simulink model "Actuatorsim"  (R2023a)
settings: Solver=FixedStepAuto  StartTime=0.0  StopTime=tf  FixedStep=tstep  RelTol=1e-3
values from neighbouring files (symbols this model uses):
  a_ol = [1 2*zeta*wn wn^2]    [ActuatorModel.m]
  b_ol = K*wn^2    (= 6103.86868538)    [ActuatorModel.m]
  k = 55    [ActuatorModel.m]    (also in SysID.m = 11.93; Translational.m = -inv(R)*Bbar'*P)
  p = -800    [ActuatorModel.m]
  z = -375    [ActuatorModel.m]
libraries: simulink x3, simulink_extras x1
settings Model: Creator=Nathan Dablain  LastModifiedBy=Nathan Dablain

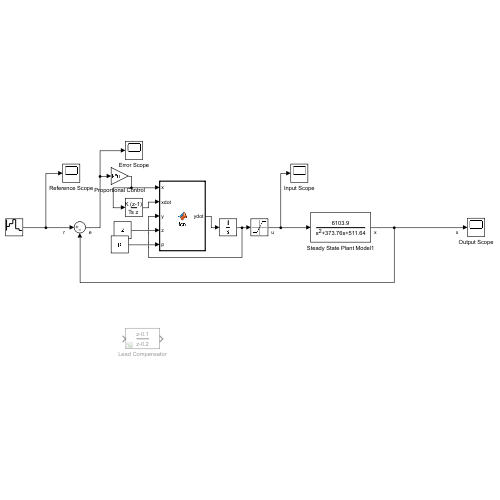
[thumbnail: Simulink's stored preview of the top-level diagram]
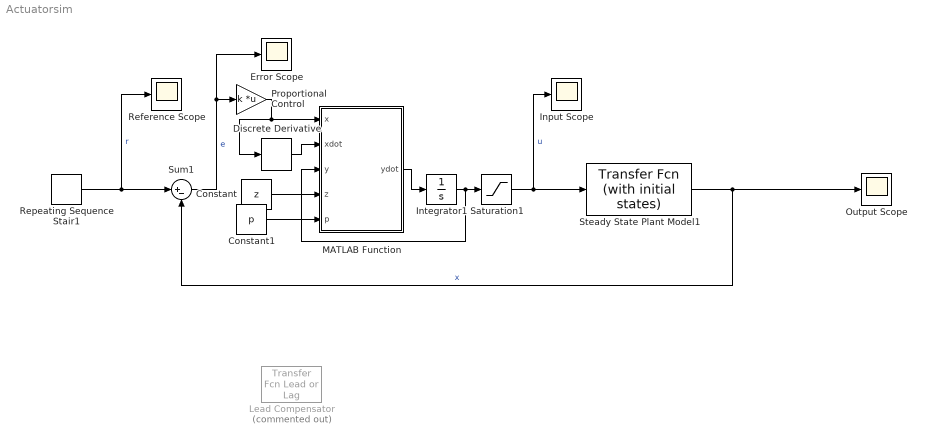
== system Actuatorsim ==
  Constant : Constant  Value=z
  Constant1 : Constant  Value=p
  Discrete Derivative : simulink/Discrete/Discrete Derivative  gainval=1.0  ICPrevScaledInput=0.0  OutMin=[]  OutMax=[]  OutDataType=fixdt(1, 16)  OutScaling=2^-10  DoSatur=off
  Error Scope : Scope
  Input Scope : Scope
  Integrator1 : Integrator
  Lead Compensator : simulink/Discrete/Transfer Fcn Lead or Lag  Commented=on  PoleZ=p  ZeroZ=z  ICPrevOutput=0.0  ICPrevInput=0.0  DoSatur=off
  MATLAB Function : MATLAB Function  TreatAsAtomicUnit=on
  Output Scope : Scope
  Proportional Control : Gain  Gain=k  Multiplication=Matrix(K*u)
  Reference Scope : Scope
  Repeating Sequence Stair1 : simulink/Sources/Repeating Sequence Stair  OutValues=[1000 1200 1427 890 777].'  tsamp=0.5  OutMin=[]  OutMax=[]  OutDataTypeStr=double  OutputDataTypeScalingMode=double  OutDataType=fixdt(0,8)  ConRadixGroup=Best Precision: Vector-wise  OutScaling=2^-12
  Saturation1 : Saturate  UpperLimit=255  LowerLimit=0
  Steady State Plant Model1 : simulink_extras/Additional Linear/Transfer Fcn (with initial states)  N=b_ol  D=a_ol  X0=0
  Sum1 : Sum  Inputs=|+-
  wires:
  Repeating Sequence Stair1/1 -> Sum1/1, Reference Scope/1  "r"
  Saturation1/1 -> Steady State Plant Model1/1, Input Scope/1  "u"
  Steady State Plant Model1/1 -> Sum1/2, Output Scope/1  "x"
  Sum1/1 -> Error Scope/1, Proportional Control/1  "e"
  Proportional Control/1 -> Discrete Derivative/1, MATLAB Function/1(x)
  MATLAB Function/1(ydot) -> Integrator1/1
  Integrator1/1 -> MATLAB Function/3(y), Saturation1/1
  Discrete Derivative/1 -> MATLAB Function/2(xdot)
  Constant1/1 -> MATLAB Function/5(p)
  Constant/1 -> MATLAB Function/4(z)

== matlab function Actuatorsim/MATLAB Function ==
  data: x input; ydot output; xdot input; y input; z input; p input
function ydot = fcn(x,xdot,y,z,p)
    ydot = xdot + p*y - z*x;
end
